simulink model "MEEN432_Project2"  (R2024b)
settings: Solver=VariableStepAuto  StartTime=0.0  StopTime=10.0  RelTol=1e-3
settings Model: Creator=jpalm  LastModifiedBy=jpalm

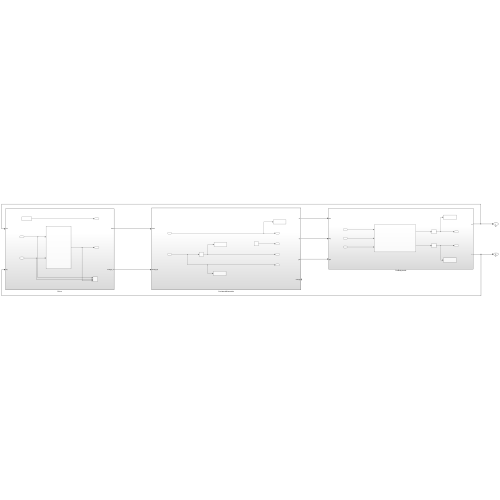
[thumbnail: Simulink's stored preview of the top-level diagram]
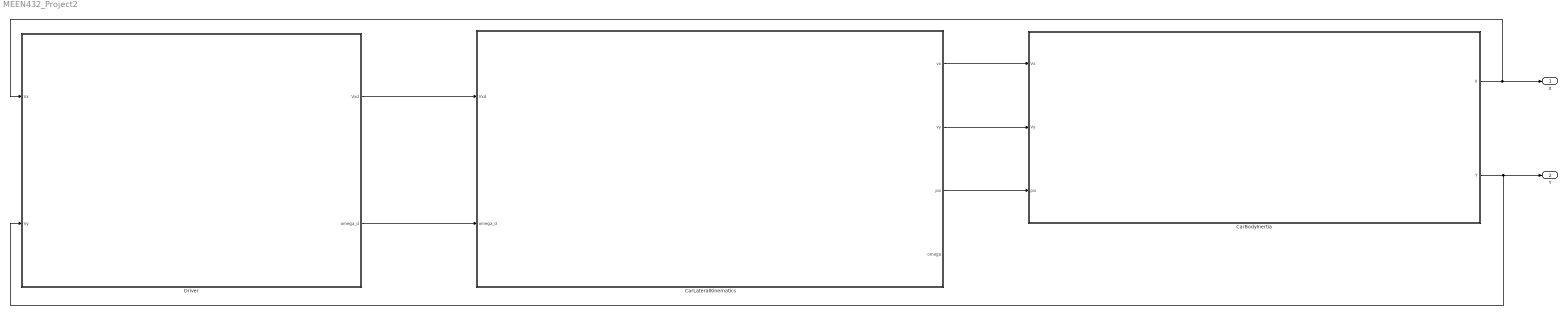
== system MEEN432_Project2 ==
  CarBodyInertia : Subsystem
  CarLateralKinematics : Subsystem
  Driver : Subsystem
  X : Outport
  Y : Outport  Port=2
  wires:
  CarBodyInertia/1(X) -> Driver/1(Vx), X/1
  CarBodyInertia/2(Y) -> Driver/2(Vy), Y/1
  CarLateralKinematics/1(vx) -> CarBodyInertia/1(Vx)
  CarLateralKinematics/2(vy) -> CarBodyInertia/2(Vy)
  CarLateralKinematics/3(psi) -> CarBodyInertia/3(psi)
  Driver/1(Vxd) -> CarLateralKinematics/1(Vxd)
  Driver/2(omega_d) -> CarLateralKinematics/2(omega_d)

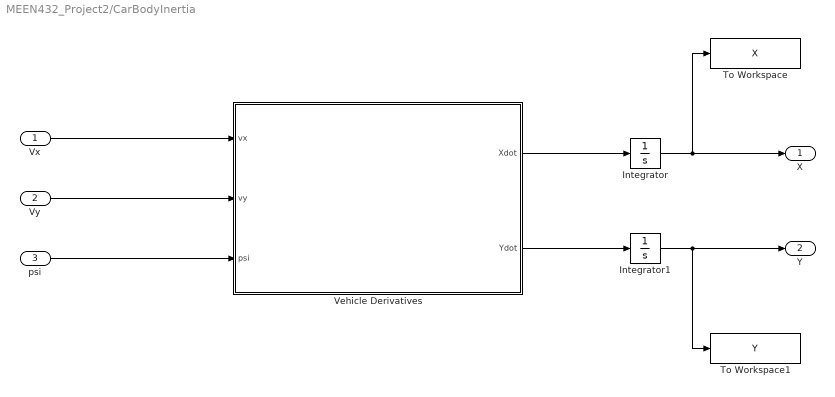
== system MEEN432_Project2/CarBodyInertia ==
  Vx : Inport
  Vy : Inport  Port=2
  psi : Inport  Port=3
  Integrator : Integrator
  Integrator1 : Integrator
  To Workspace : ToWorkspace  VariableName=X  SaveFormat=Timeseries  SampleTime=-1
  To Workspace1 : ToWorkspace  VariableName=Y  SaveFormat=Timeseries  SampleTime=-1
  Vehicle Derivatives : MATLAB Function  TreatAsAtomicUnit=on
  X : Outport
  Y : Outport  Port=2
  wires:
  Integrator/1 -> X/1, To Workspace/1
  psi/1 -> Vehicle Derivatives/3(psi)
  Integrator1/1 -> Y/1, To Workspace1/1
  Vehicle Derivatives/1(Xdot) -> Integrator/1
  Vx/1 -> Vehicle Derivatives/1(vx)
  Vy/1 -> Vehicle Derivatives/2(vy)
  Vehicle Derivatives/2(Ydot) -> Integrator1/1

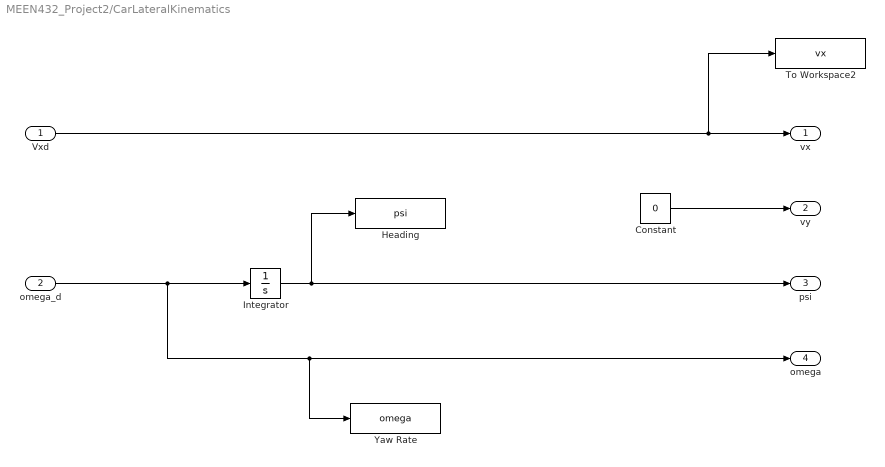
== system MEEN432_Project2/CarLateralKinematics ==
  Vxd : Inport
  omega_d : Inport  Port=2
  Constant : Constant  Value=0
  Heading : ToWorkspace  VariableName=psi  SaveFormat=Timeseries  SampleTime=-1
  Integrator : Integrator
  To Workspace2 : ToWorkspace  VariableName=vx  SaveFormat=Timeseries  SampleTime=-1
  Yaw Rate : ToWorkspace  VariableName=omega  SaveFormat=Timeseries  SampleTime=-1
  vx : Outport
  vy : Outport  Port=2
  psi : Outport  Port=3
  omega : Outport  Port=4
  wires:
  omega_d/1 -> omega/1, Yaw Rate/1, Integrator/1
  Vxd/1 -> vx/1, To Workspace2/1
  Constant/1 -> vy/1
  Integrator/1 -> Heading/1, psi/1

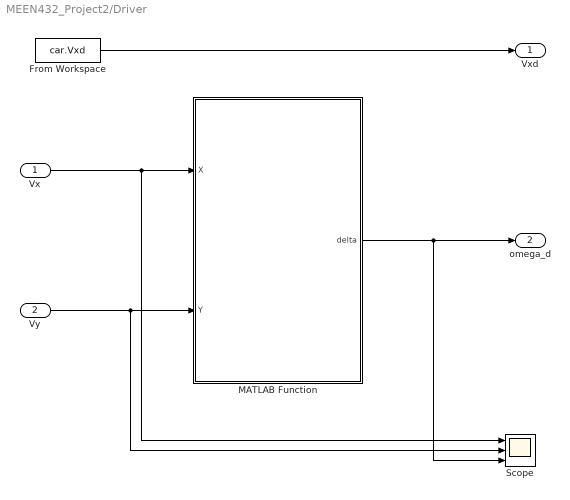
== system MEEN432_Project2/Driver ==
  Vx : Inport
  Vy : Inport  Port=2
  From Workspace : FromWorkspace  VariableName=car.Vxd
  MATLAB Function : MATLAB Function  TreatAsAtomicUnit=on
  Scope : Scope  NumInputPorts=3
  Vxd : Outport
  omega_d : Outport  Port=2
  wires:
  MATLAB Function/1(delta) -> omega_d/1, Scope/3
  Vx/1 -> Scope/1, MATLAB Function/1(X)
  Vy/1 -> Scope/2, MATLAB Function/2(Y)
  From Workspace/1 -> Vxd/1

== matlab function MEEN432_Project2/Driver/MATLAB Function ==
  data: X input; delta output; Y input
function delta = Driver(X,Y)
    if X>900
        delta = 0.5;
    elseif X < 0
        delta = 0.5;
    else
        delta = 0;
    end
end

== matlab function MEEN432_Project2/CarBodyInertia/Vehicle Derivatives ==
  data: vx input; Xdot output; vy input; psi input; Ydot output
function [Xdot, Ydot] = fcn(vx, vy, psi)
    temp = TF(psi) * [vx;vy];
    Xdot = temp(1);
    Ydot = temp(2);

end

function y = TF(psi)
    y = [cos(psi), -sin(psi); sin(psi), cos(psi)];
end
